simulink model "example1"  (Simulink 3.00)
settings: Solver=ode45  StartTime=0.0  StopTime=10.0  FixedStep=0.01  RelTol=1e-3
settings Model: LastModifiedBy=ltn100

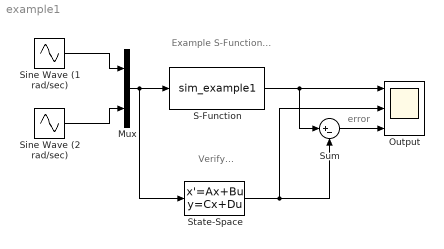
== system example1 ==
  note: Example S-Function...
  note: Verify...
  note: error
  Mux : Mux  Inputs=2
  Output : Scope  NumInputPorts=3
      settings: TimeRange=10  YMin=-4~-4~-5e-016  YMax=4~4~1.5e-015  SaveToWorkspace=off  SaveName=ScopeData
  S-Function : S-Function  FunctionName=sim_example1  PortCounts=[]  SFunctionModules=''
  Sine Wave (1 rad/sec) : Sin  Amplitude=1  Frequency=1  Phase=0  SampleTime=0
  Sine Wave (2 rad/sec) : Sin  Amplitude=1  Frequency=2  Phase=0  SampleTime=0
  State-Space : StateSpace  A=[-15 -18 0;1 0 0;0 1 0]  B=[1 0.5;0 0;0 0]  C=[8 1 0;4 5 0]  D=[-1 -2;-3 -2]  X0=[0 0 0]
  Sum : Sum  Inputs=|+-  SaturateOnIntegerOverflow=on
  wires:
  Sine Wave (2 rad/sec)/1 -> Mux/2
  Sine Wave (1 rad/sec)/1 -> Mux/1
  Mux/1 -> S-Function/1, State-Space/1
  Sum/1 -> Output/3
  S-Function/1 -> Sum/1, Output/1
  State-Space/1 -> Sum/2, Output/2
